simulink model "Esempio6_s"  (R2021b)
settings: Solver=VariableStepAuto  StartTime=0.0  StopTime=10.0  RelTol=1e-3
undefined symbols (not defined in the file): A, B, C, k1, k2
settings Model: Creator=Steph  LastModifiedBy=Steph

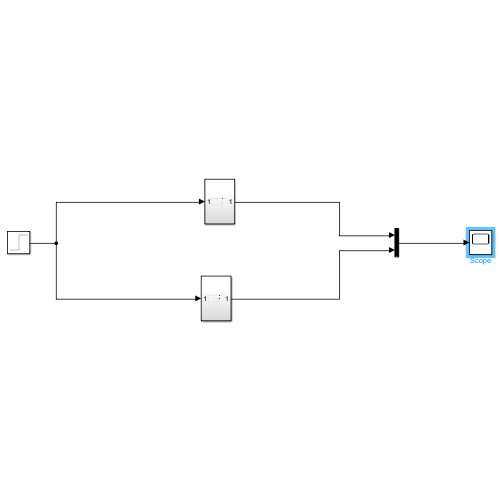
[thumbnail: Simulink's stored preview of the top-level diagram]
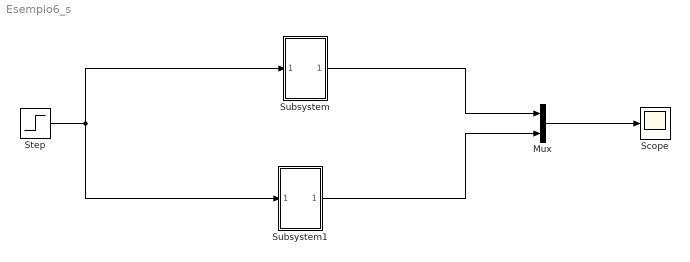
== system Esempio6_s ==
  Mux : Mux  Inputs=2
  Scope : Scope
  Step : Step  SampleTime=0
  Subsystem : Subsystem
  Subsystem1 : Subsystem
  wires:
  Mux/1 -> Scope/1
  Step/1 -> Subsystem1/1(In1), Subsystem/1(In1)
  Subsystem/1(Out1) -> Mux/1
  Subsystem1/1(Out1) -> Mux/2

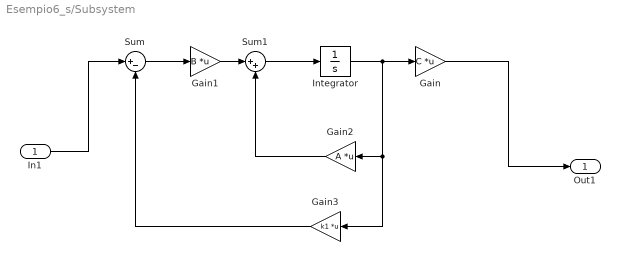
== system Esempio6_s/Subsystem ==
  In1 : Inport
  Gain : Gain  Gain=C  Multiplication=Matrix(K*u)
  Gain1 : Gain  Gain=B  Multiplication=Matrix(K*u)
  Gain2 : Gain  Gain=A  Multiplication=Matrix(K*u)
  Gain3 : Gain  Gain=k1  Multiplication=Matrix(K*u)
  Integrator : Integrator
  Sum : Sum  Inputs=|+-
  Sum1 : Sum  Inputs=|++
  Out1 : Outport
  wires:
  Gain/1 -> Out1/1
  Integrator/1 -> Gain3/1, Gain2/1, Gain/1
  Sum/1 -> Gain1/1
  Gain1/1 -> Sum1/1
  In1/1 -> Sum/1
  Gain3/1 -> Sum/2
  Gain2/1 -> Sum1/2
  Sum1/1 -> Integrator/1

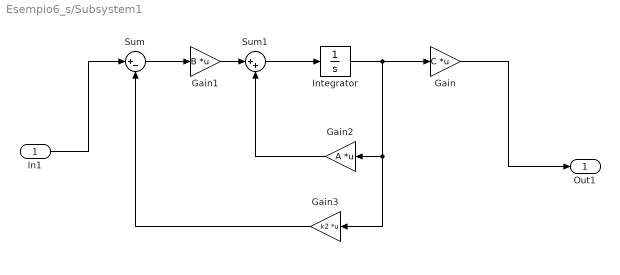
== system Esempio6_s/Subsystem1 ==
  In1 : Inport
  Gain : Gain  Gain=C  Multiplication=Matrix(K*u)
  Gain1 : Gain  Gain=B  Multiplication=Matrix(K*u)
  Gain2 : Gain  Gain=A  Multiplication=Matrix(K*u)
  Gain3 : Gain  Gain=k2  Multiplication=Matrix(K*u)
  Integrator : Integrator
  Sum : Sum  Inputs=|+-
  Sum1 : Sum  Inputs=|++
  Out1 : Outport
  wires:
  Gain/1 -> Out1/1
  Integrator/1 -> Gain3/1, Gain2/1, Gain/1
  Sum/1 -> Gain1/1
  Gain1/1 -> Sum1/1
  In1/1 -> Sum/1
  Gain3/1 -> Sum/2
  Gain2/1 -> Sum1/2
  Sum1/1 -> Integrator/1
